simulink model "p_4"  (R2018b)
settings: Solver=VariableStepAuto  StartTime=0.0  StopTime=50  MaxStep=0.01  RelTol=1e-3
settings Model: Creator=kekos  LastModifiedBy=kekos

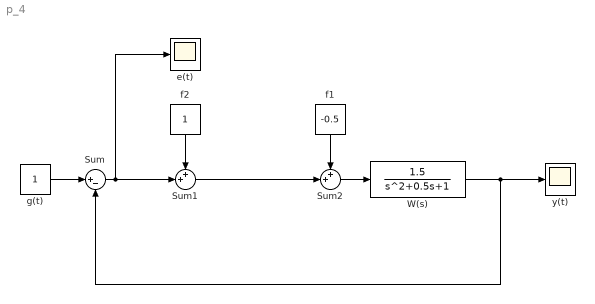
== system p_4 ==
  Sum : Sum  Inputs=|+-
  Sum1 : Sum  Inputs=++|
  Sum2 : Sum  Inputs=++|
  W(s) : TransferFcn  Numerator=[1.5]  Denominator=[1 0.5 1]
  e(t) : Scope
  f1 : Constant  Value=-0.5
  f2 : Constant
  g(t) : Constant
  y(t) : Scope
  wires:
  Sum/1 -> Sum1/2, e(t)/1
  f2/1 -> Sum1/1
  f1/1 -> Sum2/1
  Sum1/1 -> Sum2/2
  Sum2/1 -> W(s)/1
  g(t)/1 -> Sum/1
  W(s)/1 -> Sum/2, y(t)/1
